simulink model "Progetto_C1_A_sim"  (R2021a)
settings: Solver=VariableStepAuto  StartTime=0.0  StopTime=10  RelTol=1e-3
values from neighbouring files (symbols this model uses):
  beta = 1.1    [Progetto_C1_A.m]
  delta_1 = 5e4    (= 50000)    [Progetto_C1_A.m]
  delta_2 = 0.1    [Progetto_C1_A.m]
  delta_3 = 0.01    [Progetto_C1_A.m]
  gamma_1 = 0.5;,    [Progetto_C1_A.m]
  gamma_2 = 0.1    [Progetto_C1_A.m]
  gden = cell2mat(gden)    [Progetto_C1_A.m]
  gnum = cell2mat(gnum)    [Progetto_C1_A.m]
  J = 40    [Progetto_C1_A.m]
  m_e = fzero(x_2, 0)    [Progetto_C1_A.m]
  omega_e = 10    [Progetto_C1_A.m]
  psi = 0.02    [Progetto_C1_A.m]
  rden = cell2mat(rden)    [Progetto_C1_A.m]
  rnum = cell2mat(rnum)    [Progetto_C1_A.m]
  u_e = u_e_1    [Progetto_C1_A.m]
settings Model: OrderedModelArguments=off  Creator=Andrea  LastModifiedBy=Andrea

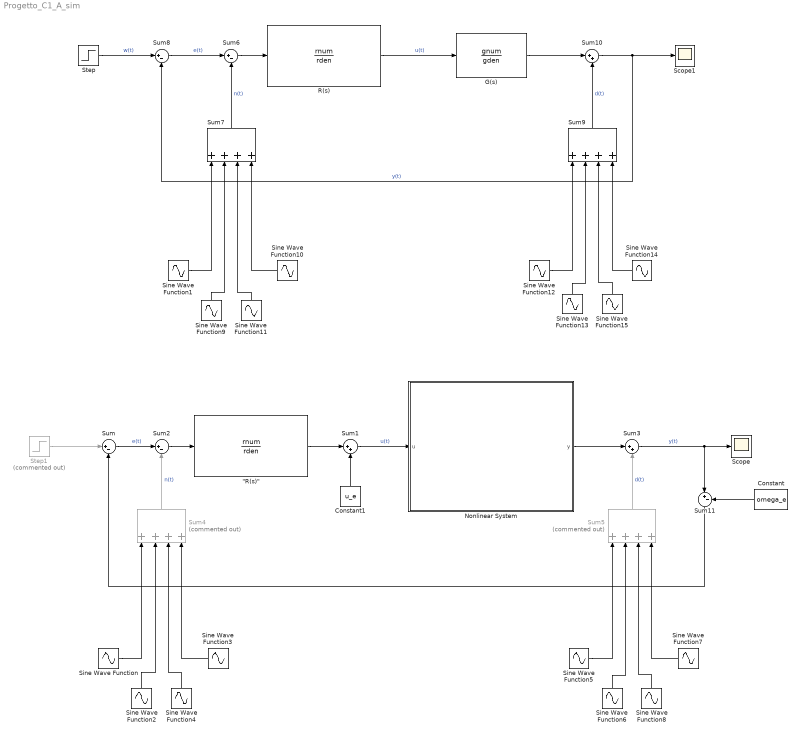
== system Progetto_C1_A_sim ==
  "\"R(s)\"" : TransferFcn  Numerator=rnum  Denominator=rden
  Constant : Constant  Value=omega_e
  Constant1 : Constant  Value=u_e
  G(s) : TransferFcn  Numerator=gnum  Denominator=gden
  Nonlinear System : Subsystem
  R(s) : TransferFcn  Numerator=rnum  Denominator=rden
  Scope : Scope
  Scope1 : Scope
  Sine Wave Function : Sin  Amplitude=0.1  Frequency=5000  SampleTime=0
  Sine Wave Function1 : Sin  Amplitude=0.1  Frequency=5000  SampleTime=0
  Sine Wave Function10 : Sin  Amplitude=0.1  Frequency=20000  SampleTime=0
  Sine Wave Function11 : Sin  Amplitude=0.1  Frequency=15000  SampleTime=0
  Sine Wave Function12 : Sin  Amplitude=0.3  Frequency=0.01875  SampleTime=0
  Sine Wave Function13 : Sin  Amplitude=0.3  Frequency=0.0375  SampleTime=0
  Sine Wave Function14 : Sin  Amplitude=0.3  Frequency=0.075  SampleTime=0
  Sine Wave Function15 : Sin  Amplitude=0.3  Frequency=0.05625  SampleTime=0
  Sine Wave Function2 : Sin  Amplitude=0.1  Frequency=10000  SampleTime=0
  Sine Wave Function3 : Sin  Amplitude=0.1  Frequency=20000  SampleTime=0
  Sine Wave Function4 : Sin  Amplitude=0.1  Frequency=15000  SampleTime=0
  Sine Wave Function5 : Sin  Amplitude=0.3  Frequency=0.01875  SampleTime=0
  Sine Wave Function6 : Sin  Amplitude=0.3  Frequency=0.0375  SampleTime=0
  Sine Wave Function7 : Sin  Amplitude=0.3  Frequency=0.075  SampleTime=0
  Sine Wave Function8 : Sin  Amplitude=0.3  Frequency=0.05625  SampleTime=0
  Sine Wave Function9 : Sin  Amplitude=0.1  Frequency=10000  SampleTime=0
  Step : Step  Time=0  After=0.5  SampleTime=0
  Step1 : Step  Commented=on  Time=0  After=0.00000682445  SampleTime=0
  Sum{,2,6,8,11} (5 alike) : Sum  Inputs=|+-
  Sum1 : Sum  Inputs=|++
  Sum10 : Sum  Inputs=|++
  Sum3 : Sum  Inputs=|++
  Sum4 : Sum  Commented=on  Inputs=++++
  Sum5 : Sum  Commented=on  Inputs=++++
  Sum7 : Sum  Inputs=++++
  Sum9 : Sum  Inputs=++++
  wires:
  Sum/1 -> Sum2/1  "e(t)"
  Constant1/1 -> Sum1/2
  Sum3/1 -> Sum11/1, Scope/1  "y(t)"
  Sum2/1 -> "\"R(s)\""/1
  Nonlinear System/1(y) -> Sum3/1
  Sum1/1 -> Nonlinear System/1(u)  "u(t)"
  Sine Wave Function/1 -> Sum4/1
  Sine Wave Function2/1 -> Sum4/2
  Sine Wave Function4/1 -> Sum4/3
  Sine Wave Function3/1 -> Sum4/4
  Sine Wave Function5/1 -> Sum5/1
  Sine Wave Function6/1 -> Sum5/2
  Sine Wave Function7/1 -> Sum5/4
  Sine Wave Function8/1 -> Sum5/3
  Sine Wave Function10/1 -> Sum7/4
  Sine Wave Function11/1 -> Sum7/3
  Sine Wave Function9/1 -> Sum7/2
  Sine Wave Function1/1 -> Sum7/1
  Sum6/1 -> R(s)/1
  Sum8/1 -> Sum6/1  "e(t)"
  Sum10/1 -> Scope1/1, Sum8/2  "y(t)"
  Sine Wave Function15/1 -> Sum9/3
  Sine Wave Function14/1 -> Sum9/4
  Sine Wave Function12/1 -> Sum9/1
  Sine Wave Function13/1 -> Sum9/2
  G(s)/1 -> Sum10/1
  "\"R(s)\""/1 -> Sum1/1
  Sum11/1 -> Sum/2
  Constant/1 -> Sum11/2
  R(s)/1 -> G(s)/1  "u(t)"
  Step/1 -> Sum8/1  "w(t)"
  Step1/1 -> Sum/1
  Sum5/1 -> Sum3/2  "d(t)"
  Sum7/1 -> Sum6/2  "n(t)"
  Sum9/1 -> Sum10/2  "d(t)"
  Sum4/1 -> Sum2/2  "n(t)"

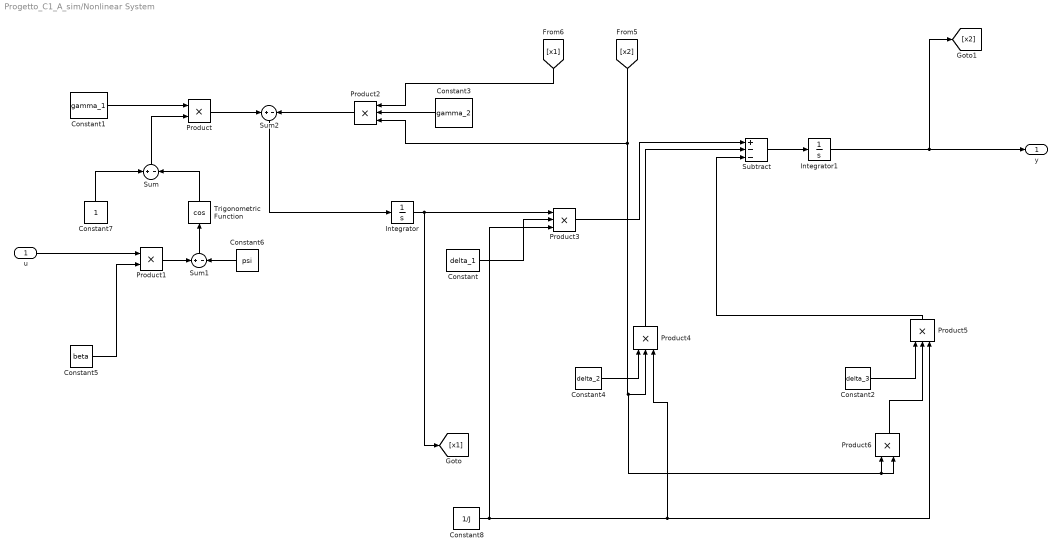
== system Progetto_C1_A_sim/Nonlinear System ==
  u : Inport
  Constant : Constant  Value=delta_1
  Constant1 : Constant  Value=gamma_1
  Constant2 : Constant  Value=delta_3
  Constant3 : Constant  Value=gamma_2
  Constant4 : Constant  Value=delta_2
  Constant5 : Constant  Value=beta
  Constant6 : Constant  Value=psi
  Constant7 : Constant
  Constant8 : Constant  Value=1/J
  Integrator : Integrator  InitialCondition=m_e  ZeroCross=off
  Integrator1 : Integrator  InitialCondition=omega_e  ZeroCross=off
  Product : Product
  Product1 : Product
  Product{2..5} (4 alike) : Product  Inputs=3
  Product6 : Product
  Subtract : Sum  Inputs=+--
  Sum : Sum  Inputs=+-
  Sum1 : Sum  Inputs=+-
  Sum2 : Sum  Inputs=+-
  Trigonometric Function : Trigonometry  Operator=cos
  y : Outport
  wires:
  Constant1/1 -> Product/1
  Sum/1 -> Product/2
  Constant7/1 -> Sum/1
  Trigonometric Function/1 -> Sum/2
  Sum1/1 -> Trigonometric Function/1
  Constant6/1 -> Sum1/2
  Product1/1 -> Sum1/1
  Constant5/1 -> Product1/2
  u/1 -> Product1/1
  Product/1 -> Sum2/1
  Product2/1 -> Sum2/2
  [x1] -> Product2/1
  Constant3/1 -> Product2/2
  Sum2/1 -> Integrator/1
  Integrator/1 -> Product3/1, [x1]
  Constant8/1 -> Product4/3, Product5/3, Product3/3
  Constant/1 -> Product3/2
  Constant4/1 -> Product4/1
  Constant2/1 -> Product5/1
  Product6/1 -> Product5/2
  Integrator1/1 -> [x2], y/1
  [x2] -> Product2/3, Product6/1, Product6/2, Product4/2
  Subtract/1 -> Integrator1/1
  Product3/1 -> Subtract/1
  Product4/1 -> Subtract/2
  Product5/1 -> Subtract/3
